simulink model "Proportional_ZOH"  (R2020b)
settings: Solver=VariableStepAuto  StartTime=0.0  StopTime=3  RelTol=1e-3
values from neighbouring files (symbols this model uses):
  T = 0.0325    [PID Katsayilari.m]
undefined symbols (not defined in the file or in its folder): DiscIntNeverNeededParam, kd, ki, kp
libraries: simulink x1
settings Model: Creator=HCS  LastModifiedBy=HCS

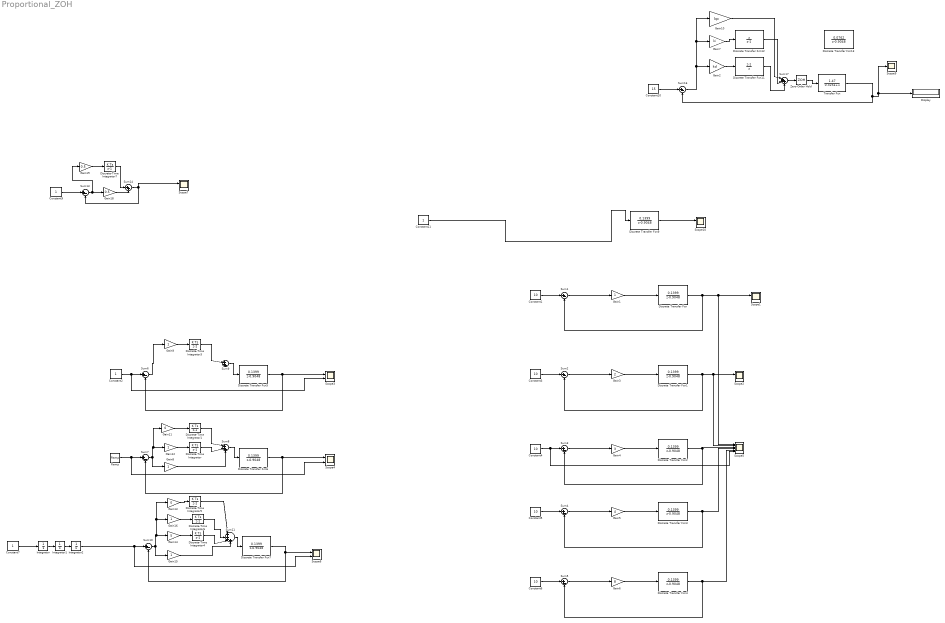
== system Proportional_ZOH ==
  Constant{1,3..6} (5 alike) : Constant  Value=10
  Constant10 : Constant  Value=15
  Constant{2,7,9,11} (4 alike) : Constant
  Discrete Transfer Fcn{,1..7,9} (9 alike) : DiscreteTransferFcn  Numerator=[0.1399]  Denominator=[1 -0.9048]
  Discrete Transfer Fcn11 : DiscreteTransferFcn  Numerator=[1 -1]  Denominator=[1 0]
  Discrete Transfer Fcn12 : DiscreteTransferFcn  Numerator=[1 0]  Denominator=[1 -1]
  Discrete Transfer Fcn13 : DiscreteTransferFcn  Numerator=[0.0762]  Denominator=[1 -0.9048]
  Discrete-Time Integrator{,1,3..7} (7 alike) : DiscreteIntegrator  SampleTime=-1  ICPrevOutput=DiscIntNeverNeededParam  ICPrevScaledInput=DiscIntNeverNeededParam
  Display : Display
  Gain{1,8..9,12,15..16} (6 alike) : Gain
  Gain10 : Gain  Gain=kp
  Gain11 : Gain  Gain=0
  Gain13 : Gain  Gain=0
  Gain14 : Gain  Gain=5
  Gain18 : Gain  Gain=0.5
  Gain19 : Gain  Gain=0.5
  Gain2 : Gain  Gain=kd
  Gain3 : Gain  Gain=2
  Gain4 : Gain  Gain=3
  Gain5 : Gain  Gain=4
  Gain6 : Gain  Gain=8
  Gain7 : Gain  Gain=ki
  Integrator : Integrator
  Integrator1 : Integrator
  Integrator2 : Integrator
  Ramp : simulink/Sources/Ramp  slope=1  start=0  InitialOutput=0
  Scope{1..4,6..7,10} (7 alike) : Scope  NumInputPorts=2
  Scope5 : Scope  NumInputPorts=6
  Scope9 : Scope
  Sum{1..7,10,13,16} (10 alike) : Sum  Inputs=|+-
  Sum11 : Sum  Inputs=|++++
  Sum14 : Sum  Inputs=|++
  Sum17 : Sum  Inputs=|+++
  Sum8 : Sum  Inputs=|+++
  Sum9 : Sum  Inputs=|+++
  Transfer Fcn : TransferFcn  Numerator=[1.47]  Denominator=[0.325 1]
  Zero-Order Hold : ZeroOrderHold  SampleTime=T
  wires:
  Sum1/1 -> Gain1/1
  Constant1/1 -> Sum1/1
  Gain1/1 -> Discrete Transfer Fcn/1
  Discrete Transfer Fcn1/1 -> Scope5/2, Scope2/1, Sum2/2
  Gain3/1 -> Discrete Transfer Fcn1/1
  Constant3/1 -> Sum2/1
  Sum2/1 -> Gain3/1
  Gain4/1 -> Discrete Transfer Fcn2/1
  Discrete Transfer Fcn2/1 -> Scope5/3, Sum3/2
  Sum3/1 -> Gain4/1
  Constant5/1 -> Sum4/1
  Gain5/1 -> Discrete Transfer Fcn3/1
  Discrete Transfer Fcn3/1 -> Scope5/4, Sum4/2
  Sum4/1 -> Gain5/1
  Discrete Transfer Fcn/1 -> Scope5/1, Scope1/1, Sum1/2
  Constant6/1 -> Sum5/1
  Gain6/1 -> Discrete Transfer Fcn4/1
  Sum5/1 -> Gain6/1
  Discrete Transfer Fcn4/1 -> Scope5/5, Sum5/2
  Constant2/1 -> Scope3/2, Sum6/1
  Discrete Transfer Fcn5/1 -> Scope3/1, Sum6/2
  Discrete Transfer Fcn6/1 -> Scope4/1, Sum7/2
  Ramp/1 -> Scope4/2, Sum7/1
  Sum7/1 -> Gain11/1, Gain12/1, Gain8/1
  Sum8/1 -> Discrete Transfer Fcn6/1
  Gain8/1 -> Sum8/3
  Discrete-Time Integrator/1 -> Sum8/2
  Discrete-Time Integrator1/1 -> Sum8/1
  Discrete-Time Integrator3/1 -> Sum9/1
  Sum6/1 -> Gain9/1
  Sum9/1 -> Discrete Transfer Fcn5/1
  Gain9/1 -> Discrete-Time Integrator3/1
  Gain11/1 -> Discrete-Time Integrator1/1
  Gain12/1 -> Discrete-Time Integrator/1
  Discrete-Time Integrator5/1 -> Sum11/1
  Gain15/1 -> Sum11/4
  Discrete Transfer Fcn7/1 -> Sum10/2, Scope6/1
  Gain13/1 -> Discrete-Time Integrator5/1
  Sum11/1 -> Discrete Transfer Fcn7/1
  Gain14/1 -> Discrete-Time Integrator4/1
  Discrete-Time Integrator4/1 -> Sum11/3
  Integrator2/1 -> Scope6/2, Sum10/1
  Integrator/1 -> Integrator1/1
  Integrator1/1 -> Integrator2/1
  Constant7/1 -> Integrator/1
  Constant4/1 -> Scope5/6, Sum3/1
  Gain16/1 -> Discrete-Time Integrator6/1
  Discrete-Time Integrator6/1 -> Sum11/2
  Sum10/1 -> Gain16/1, Gain13/1, Gain14/1, Gain15/1
  Sum13/1 -> Gain19/1, Gain18/1
  Gain19/1 -> Discrete-Time Integrator7/1
  Constant9/1 -> Sum13/1
  Gain18/1 -> Sum14/2
  Discrete-Time Integrator7/1 -> Sum14/1
  Sum14/1 -> Scope7/1, Sum13/2
  Discrete Transfer Fcn9/1 -> Scope10/1
  Constant11/1 -> Discrete Transfer Fcn9/1
  Zero-Order Hold/1 -> Transfer Fcn/1
  Sum16/1 -> Gain10/1, Gain7/1, Gain2/1
  Sum17/1 -> Zero-Order Hold/1
  Transfer Fcn/1 -> Scope9/1, Display/1, Sum16/2
  Gain10/1 -> Sum17/1
  Discrete Transfer Fcn12/1 -> Sum17/2
  Discrete Transfer Fcn11/1 -> Sum17/3
  Gain7/1 -> Discrete Transfer Fcn12/1
  Gain2/1 -> Discrete Transfer Fcn11/1
  Constant10/1 -> Sum16/1
